simulink model "PlanningSubsystem"  (R2019b)
settings: Solver=VariableStepAuto  StartTime=0.0  StopTime=10.0  RelTol=1e-3
settings Model: Creator=loker  LastModifiedBy=loker

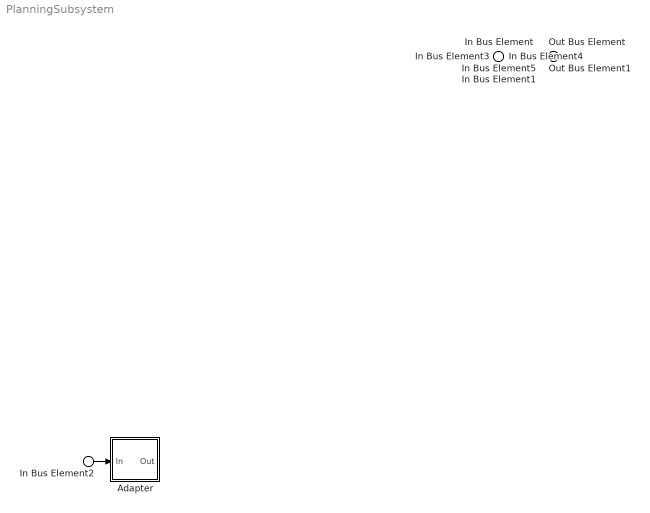
== system PlanningSubsystem ==
  In Bus Element5 : Inport  PortName=Trajectory Predictions
  In Bus Element : Inport  Port=2  PortName=Lidar Data
  In Bus Element1 : Inport  Port=3  PortName=IMU Data
  In Bus Element2 : Inport  Port=4  PortName=Wheel State Data
  In Bus Element3 : Inport  Port=5  PortName=Environment Map
  In Bus Element4 : Inport  Port=6  PortName=Task
  Adapter : Subsystem
      settings: PortSchema="{\"entries\":[{\"content\":{\"margin\":10,\"minimumSpacing\":10,\"sides\":[{\"content\":{\"connectorIds\":[\"In1\"]},\"type\":\"ConnectorPlacement.EquallySpacedRectSide\",\"uuid\":\"9c658e47-9141-4b09-899d-e7d6eeef288e\"},{\"content\":{\"connectorIds\":[\"Out1\"],\"side\":\"RIGHT\"},\"type\":\"ConnectorPlacement.EquallySpacedRectSide\",\"uuid\":\"7a582264-0565-42d4-adb3-e560ad597e55\"},{\"content\":{\"connectorIds\":[],\"side\":\"TOP\"},\"type\":\"ConnectorPlacement.EquallySpacedRectSide\",\"uuid\":\"701b4c6c-e203-4bd7-b8b7-cb8feb01699c\"}]},\"type\":\"ConnectorPlacement.EquallySpacedConnector\",\"uuid\":\"2059a5e9-c0d5-4fb6-87cf-b1bfdc666ab8\"}],\"packageUris\":[\"http://schema.mathworks.com/mf0/Connector/19700101\"],\"version\":\"1.0\"}"
  Out Bus Element1 : Outport  PortName=Planned Trajectory
  Out Bus Element : Outport  Port=2  PortName=Desired Wheel State
  wires:
  In Bus Element2/1 -> Adapter/1(In)

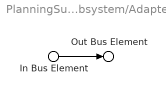
== system PlanningSubsystem/Adapter ==
  In Bus Element : Inport  PortName=In
  Out Bus Element : Outport  PortName=Out
  wires:
  In Bus Element/1 -> Out Bus Element/1
